simulink model "pglib"  (Simulink 7.0)
settings: Solver=ode45  SolverMode=SingleTasking  StartTime=0.0  StopTime=10.0  RelTol=1e-3  AbsTol=1e-6
(part 1 of 3)
settings Model: Creator=jacobs  LastModifiedBy=lfd  ExtModeAutoUpdateStatusClock=off
settings DataIOCC: LimitDataPoints=off
settings OptimizationCC: BlockReduction=off  BooleanDataType=off
settings DebuggingCC: SaveWithParameterizedLinksMsg=none  SignalResolutionControl=TryResolveAllWithWarning  SolverPrmCheckMsg=none  MultiTaskDSMMsg=warning  MultiTaskCondExecSysMsg=none  StrictBusMsg=None
settings HardwareCC: TargetUnknown=on
settings RTWCC: IncludeERTFirstTime=on
settings GRTTargetCC: TargetFcnLib=ansi_tfl_tmw.mat  ModelReferenceCompliant=off  MatFileLogging=off

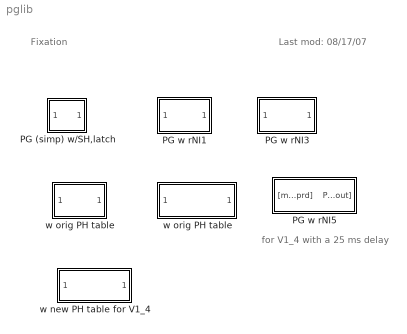
== system pglib ==
  note: Last mod: 08/17/07
  note: Fixation
  note: for V1_4 with a 25 ms delay
  PG (simp) w/SH,latch : Subsystem
      mask Display: disp('PG')
  PG w rNI1 : Subsystem
      mask Display: disp('PG rNI 1\n(2P)')
  PG w rNI3 : Subsystem
      mask Display: disp('PG rNI 1ltnl\n(2P)')
  PG w rNI5 : Subsystem
      mask Display: disp('PG25 rNI V1_4\n(2P)')
  w new PH table for V1_4 : Subsystem
      mask Display: disp('PG rNI V1_4\n(2P)')
  w orig PH table : Subsystem
      mask Display: disp('PG rNI 2\n(2P)')
  "w orig PH table  " : Subsystem
      mask Display: disp('PG rNI V1_4\n(2P)')

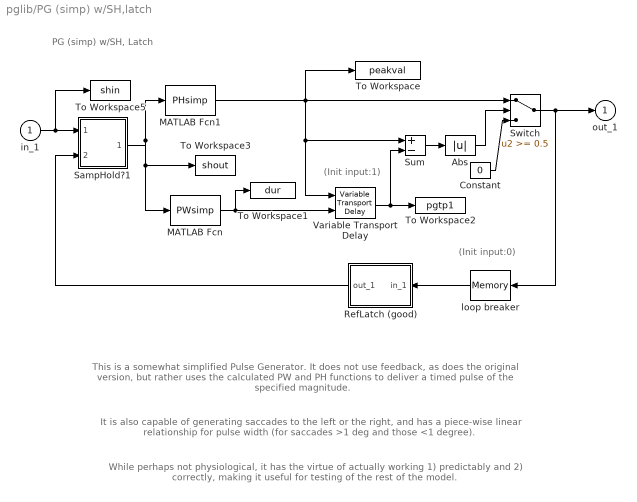
== system pglib/PG (simp) w/SH,latch ==
  note: (Init input:0)
  note: (Init input:1)
  note: PG (simp) w/SH, Latch
  note: This is a somewhat simplified Pulse Generator.  It does not use feedback, as does the
      | original version, but rather uses the calculated PW and PH functions to deliver
      | a timed pulse of the specified magnitude.
  note: It is also capable of generating saccades to the left or the right, and has a piece-wise
      | linear relationship for pulse width (for saccades >1 deg and those <1 degree).
  note: While perhaps not physiological, it has the virtue of actually working
      | 1) predictably and 2) correctly, making it useful for testing of the rest of the model.
  in_1 : Inport  OutDataType=sfix(16)  OutScaling=2^0
  Abs : Abs  SaturateOnIntegerOverflow=on
  Constant : Constant  Value=0  OutDataType=sfix(16)  OutScaling=2^0
  MATLAB Fcn : MATLABFcn  MATLABFcn=PWsimp
      mask Help: u>=1: y=(1.3*abs(u)+12)/1000\nu <1: y=(12*abs(u))/1000
      mask Display: disp('PW\nsimp')
  MATLAB Fcn1 : MATLABFcn  MATLABFcn=PHsimp
      mask Help: u<=0.25: y=0\nu> 0.25:  y = 590*u/(7.5+abs(u))
      mask Display: disp('PH\nsimp')
  RefLatch (good) : Subsystem  Orientation=left  mask{@1=50}
      mask prompts: @1 "Refractory Period (ms)"
      mask help: Refractory Latch
      mask init:
      | delay=@1;
      mask Display: disp('Refract\nLatch')
  SampHold?1 : Subsystem
      mask Display: disp('S&H\n(S=H)\n(H=L)')
  Sum : Sum  Inputs=+-  OutDataType=sfix(16)  OutScaling=2^0  SaturateOnIntegerOverflow=on  InputSameDT=on
  Switch : Switch  Threshold=0.5  SaturateOnIntegerOverflow=on  InputSameDT=on
  To Workspace : ToWorkspace  VariableName=peakval  SaveFormat=Array
      settings: MaxDataPoints=10000
  To Workspace1 : ToWorkspace  VariableName=dur  SaveFormat=Array
      settings: MaxDataPoints=10000
  To Workspace2 : ToWorkspace  VariableName=pgtp1  SaveFormat=Array
      settings: MaxDataPoints=10000
  To Workspace3 : ToWorkspace  VariableName=shout  SaveFormat=Array
      settings: MaxDataPoints=10000
  To Workspace5 : ToWorkspace  VariableName=shin  SaveFormat=Array
      settings: MaxDataPoints=10000
  Variable Transport Delay : VariableTransportDelay  MaximumDelay=10  InitialOutput=1
  loop breaker : Memory  Orientation=left
  out_1 : Outport  OutDataType=sfix(16)  OutScaling=2^0  InitialOutput=0
  wires:
  RefLatch (good)/1(out_1) -> SampHold?1/2(S/H?)
  SampHold?1/1(output) -> To Workspace3/1, MATLAB Fcn/1, MATLAB Fcn1/1
  in_1/1 -> To Workspace5/1, SampHold?1/1(Input)
  MATLAB Fcn1/1 -> To Workspace/1, Sum/1, Variable Transport Delay/1, Switch/1
  Switch/1 -> out_1/1, loop breaker/1
  Constant/1 -> Switch/3
  Variable Transport Delay/1 -> Sum/2, To Workspace2/1
  loop breaker/1 -> RefLatch (good)/1(in_1)
  Abs/1 -> Switch/2
  Sum/1 -> Abs/1
  MATLAB Fcn/1 -> To Workspace1/1, Variable Transport Delay/2

== system pglib/PG w rNI1 ==
  note: (Init input:0)
  note: PG with Resettable NI
  note: The refractory latch prevents the pulse generator from responding to another stimulus until a
      | physiologically acceptable refractory period has elapsed by controlling the "Sample and Hold" block.
  note: Here it is at last!  A pulse generator based on a resettable integrator (look inside the PW
      | block).  The PW function controls the switch, allowing the output of the PH function to pass
      | for the appropriate duration.
  "[mcsprd]" : Inport  OutDataType=sfix(16)  OutScaling=2^0
  Constant1 : Constant  Orientation=up  Value=0  OutDataType=sfix(16)  OutScaling=2^0
  PH funct : MATLABFcn  MATLABFcn=phfn_ss
      mask Display: disp('PH\nfunction')
  PW funct : Subsystem
      mask Display: disp('PW\nfunction')
  RefLatch (Default = 50ms) : Subsystem  Orientation=left  mask{@1=50}
      mask prompts: @1 "Refractory Period (ms)"
      mask help: Refractory Latch
      mask init:
      | delay=@1;
      mask Display: disp('Refract\nLatch')
  SampHold?1 : Subsystem
      mask Display: disp('S=H\nH=L')
  Switch : Switch  Threshold=0.5  SaturateOnIntegerOverflow=on  InputSameDT=on
  loop breaker : Memory  Orientation=left
  PG [pgout] : Outport  OutDataType=sfix(16)  OutScaling=2^0  InitialOutput=0
  wires:
  RefLatch (Default = 50ms)/1(out_1) -> SampHold?1/2(S/H?)
  PH funct/1 -> Switch/1
  PW funct/1(pgw) -> Switch/2
  "[mcsprd]"/1 -> SampHold?1/1(Input)
  SampHold?1/1(output) -> PW funct/1(mcspl), PH funct/1
  loop breaker/1 -> RefLatch (Default = 50ms)/1(in_1)
  Switch/1 -> PG [pgout]/1, loop breaker/1
  Constant1/1 -> Switch/3

== system pglib/PG w rNI3 ==
  note: (Init input:0)
  note: PG with Resettable NI
  note: The refractory latch prevents the pulse generator from responding to another stimulus until a
      | physiologically acceptable refractory period has elapsed by controlling the "Sample and Hold" block.
  note: Here it is at last!  A pulse generator based on a resettable integrator (look inside the PW
      | block).  The PW function controls the switch, allowing the output of the PH function to pass
      | for the appropriate duration.
  "[mcsprd]" : Inport  OutDataType=sfix(16)  OutScaling=2^0
  Constant1 : Constant  Orientation=up  Value=0  OutDataType=sfix(16)  OutScaling=2^0
  PH funct : MATLABFcn  MATLABFcn=phfn_ss
      mask Display: disp('PH\nfunction')
  PW funct : Subsystem
      mask Display: disp('PW\nfunction')
  RefLatch (Default = 50ms) : Subsystem  Orientation=left  mask{@1=50}
      mask prompts: @1 "Refractory Period (ms)"
      mask help: Refractory Latch
      mask init:
      | delay=@1;
      mask Display: disp('Refract\nLatch')
  SampHold?1 : Subsystem
      mask Display: disp('S=H\nH=L')
  Switch : Switch  Threshold=0.5  SaturateOnIntegerOverflow=on  InputSameDT=on
  loop breaker : Memory  Orientation=left
  PG [pgout] : Outport  OutDataType=sfix(16)  OutScaling=2^0  InitialOutput=0
  wires:
  RefLatch (Default = 50ms)/1(out_1) -> SampHold?1/2(S/H?)
  PH funct/1 -> Switch/1
  PW funct/1(pgw) -> Switch/2
  "[mcsprd]"/1 -> SampHold?1/1(Input)
  SampHold?1/1(output) -> PW funct/1(mcspl), PH funct/1
  loop breaker/1 -> RefLatch (Default = 50ms)/1(in_1)
  Switch/1 -> PG [pgout]/1, loop breaker/1
  Constant1/1 -> Switch/3

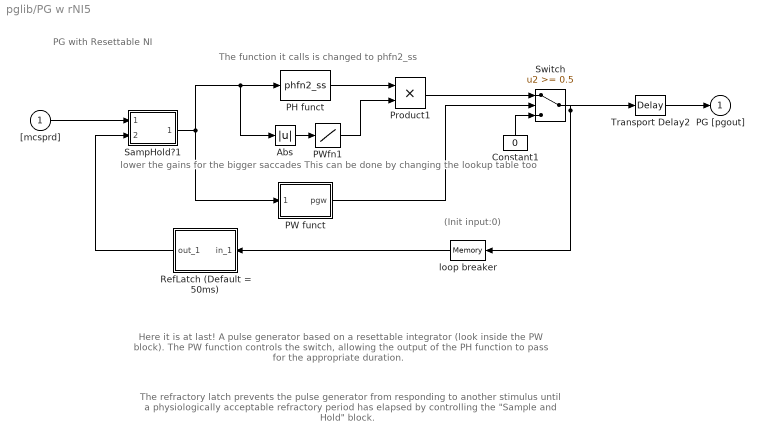
== system pglib/PG w rNI5 ==
  note: (Init input:0)
  note: PG with Resettable NI
  note: The refractory latch prevents the pulse generator from responding to another stimulus until a
      | physiologically acceptable refractory period has elapsed by controlling the "Sample and Hold" block.
  note: Here it is at last!  A pulse generator based on a resettable integrator (look inside the PW
      | block).  The PW function controls the switch, allowing the output of the PH function to pass
      | for the appropriate duration.
  note: lower the gains for the bigger saccades
      | This can be done by changing the lookup table too
  note: The function it calls is changed to phfn2_ss
  "[mcsprd]" : Inport  OutDataType=sfix(16)  OutScaling=2^0
  Abs : Abs  SaturateOnIntegerOverflow=on
  Constant1 : Constant  Orientation=up  Value=0  OutDataType=sfix(16)  OutScaling=2^0
  PH funct : MATLABFcn  MATLABFcn=phfn2_ss
      mask Display: disp('PH\nfunction')
  PW funct : Subsystem
      mask Display: disp('PW\nfunction')
  PWfn1 : Lookup  InputValues=[ 0, 0.1:20, 20:50 ]  Table="[ 0, (0.1:20)*0+1,  (20:50)*0+0.95]"  OutDataType=sfix(16)  OutScaling=2^0  SaturateOnIntegerOverflow=on
  Product1 : Product  OutDataType=sfix(16)  OutScaling=2^0  SaturateOnIntegerOverflow=on  RndMeth=Zero  InputSameDT=on
  RefLatch (Default = 50ms) : Subsystem  Orientation=left  mask{@1=50}
      mask prompts: @1 "Refractory Period (ms)"
      mask help: Refractory Latch
      mask init:
      | delay=@1;
      mask Display: disp('Refract\nLatch')
  SampHold?1 : Subsystem
      mask Display: disp('S=H\nH=L')
  Switch : Switch  Threshold=0.5  SaturateOnIntegerOverflow=on  InputSameDT=on
  Transport Delay2 : TransportDelay  DelayTime=0.025
      mask Display: disp('25ms')
  loop breaker : Memory  Orientation=left
  PG [pgout] : Outport  OutDataType=sfix(16)  OutScaling=2^0  InitialOutput=0
  wires:
  RefLatch (Default = 50ms)/1(out_1) -> SampHold?1/2(S/H?)
  PH funct/1 -> Product1/1
  PW funct/1(pgw) -> Switch/2
  "[mcsprd]"/1 -> SampHold?1/1(Input)
  SampHold?1/1(output) -> PW funct/1(mcspl), PH funct/1, Abs/1
  loop breaker/1 -> RefLatch (Default = 50ms)/1(in_1)
  Switch/1 -> loop breaker/1, Transport Delay2/1
  Constant1/1 -> Switch/3
  Transport Delay2/1 -> PG [pgout]/1
  Product1/1 -> Switch/1
  PWfn1/1 -> Product1/2
  Abs/1 -> PWfn1/1

== system pglib/w new PH table for V1_4 ==
  note: Here it is at last!  A pulse generator based on a resettable integrator (look inside the PW
      | block).  The PW function controls the switch, allowing the output of the PH function to pass
      | for the appropriate duration.
  note: The refractory latch prevents the pulse generator from responding to another stimulus until a
      | physiologically acceptable refractory period has elapsed by controlling the "Sample and Hold" block.
  note: PG with Resettable NI
  note: (Init input:0)
  "[mcsprd]" : Inport  OutDataType=sfix(16)  OutScaling=2^0
  Constant1 : Constant  Orientation=up  Value=0  OutDataType=sfix(16)  OutScaling=2^0
  PH funct : MATLABFcn  MATLABFcn=phfn2_ss
      mask Display: disp('PH\nfunction')
  PW funct : Subsystem
      mask Display: disp('PW\nfunction')
  RefLatch (Default = 50ms) : Subsystem  Orientation=left  mask{@1=50}
      mask prompts: @1 "Refractory Period (ms)"
      mask help: Refractory Latch
      mask init:
      | delay=@1;
      mask Display: disp('Refract\nLatch')
  SampHold?1 : Subsystem
      mask Display: disp('S=H\nH=L')
  Switch : Switch  Threshold=0.5  SaturateOnIntegerOverflow=on  InputSameDT=on
  loop breaker : Memory  Orientation=left
  PG [pgout] : Outport  OutDataType=sfix(16)  OutScaling=2^0  InitialOutput=0
  wires:
  Constant1/1 -> Switch/3
  Switch/1 -> loop breaker/1, PG [pgout]/1
  loop breaker/1 -> RefLatch (Default = 50ms)/1(in_1)
  SampHold?1/1(output) -> PH funct/1, PW funct/1(mcspl)
  "[mcsprd]"/1 -> SampHold?1/1(Input)
  PW funct/1(pgw) -> Switch/2
  PH funct/1 -> Switch/1
  RefLatch (Default = 50ms)/1(out_1) -> SampHold?1/2(S/H?)

== system pglib/w orig PH table ==
  note: (Init input:0)
  note: PG with Resettable NI
  note: The refractory latch prevents the pulse generator from responding to another stimulus until a
      | physiologically acceptable refractory period has elapsed by controlling the "Sample and Hold" block.
  note: Here it is at last!  A pulse generator based on a resettable integrator (look inside the PW
      | block).  The PW function controls the switch, allowing the output of the PH function to pass
      | for the appropriate duration.
  "[mcsprd]" : Inport  OutDataType=sfix(16)  OutScaling=2^0
  Constant1 : Constant  Orientation=up  Value=0  OutDataType=sfix(16)  OutScaling=2^0
  PH funct : MATLABFcn  MATLABFcn=phfn_ss
      mask Display: disp('PH\nfunction')
  PW funct : Subsystem
      mask Display: disp('PW\nfunction')
  RefLatch (Default = 50ms) : Subsystem  Orientation=left  mask{@1=50}
      mask prompts: @1 "Refractory Period (ms)"
      mask help: Refractory Latch
      mask init:
      | delay=@1;
      mask Display: disp('Refract\nLatch')
  SampHold?1 : Subsystem
      mask Display: disp('S=H\nH=L')
  Switch : Switch  Threshold=0.5  SaturateOnIntegerOverflow=on  InputSameDT=on
  loop breaker : Memory  Orientation=left
  PG [pgout] : Outport  OutDataType=sfix(16)  OutScaling=2^0  InitialOutput=0
  wires:
  RefLatch (Default = 50ms)/1(out_1) -> SampHold?1/2(S/H?)
  PH funct/1 -> Switch/1
  PW funct/1(pgw) -> Switch/2
  "[mcsprd]"/1 -> SampHold?1/1(Input)
  SampHold?1/1(output) -> PW funct/1(mcspl), PH funct/1
  loop breaker/1 -> RefLatch (Default = 50ms)/1(in_1)
  Switch/1 -> PG [pgout]/1, loop breaker/1
  Constant1/1 -> Switch/3

== system pglib/w orig PH table   ==
  note: Here it is at last!  A pulse generator based on a resettable integrator (look inside the PW
      | block).  The PW function controls the switch, allowing the output of the PH function to pass
      | for the appropriate duration.
  note: The refractory latch prevents the pulse generator from responding to another stimulus until a
      | physiologically acceptable refractory period has elapsed by controlling the "Sample and Hold" block.
  note: PG with Resettable NI
  note: (Init input:0)
  "[mcsprd]" : Inport  OutDataType=sfix(16)  OutScaling=2^0
  Constant1 : Constant  Orientation=up  Value=0  OutDataType=sfix(16)  OutScaling=2^0
  PH funct : MATLABFcn  MATLABFcn=phfn_ss
      mask Display: disp('PH\nfunction')
  PW funct : Subsystem
      mask Display: disp('PW\nfunction')
  RefLatch (Default = 50ms) : Subsystem  Orientation=left  mask{@1=50}
      mask prompts: @1 "Refractory Period (ms)"
      mask help: Refractory Latch
      mask init:
      | delay=@1;
      mask Display: disp('Refract\nLatch')
  SampHold?1 : Subsystem
      mask Display: disp('S=H\nH=L')
  Switch : Switch  Threshold=0.5  SaturateOnIntegerOverflow=on  InputSameDT=on
  loop breaker : Memory  Orientation=left
  PG [pgout] : Outport  OutDataType=sfix(16)  OutScaling=2^0  InitialOutput=0
  wires:
  Constant1/1 -> Switch/3
  Switch/1 -> loop breaker/1, PG [pgout]/1
  loop breaker/1 -> RefLatch (Default = 50ms)/1(in_1)
  SampHold?1/1(output) -> PH funct/1, PW funct/1(mcspl)
  "[mcsprd]"/1 -> SampHold?1/1(Input)
  PW funct/1(pgw) -> Switch/2
  PH funct/1 -> Switch/1
  RefLatch (Default = 50ms)/1(out_1) -> SampHold?1/2(S/H?)

== system pglib/PG (simp) w/SH,latch/RefLatch (good) ==
  note: It's a cheap trick, but it seems to work:
  note: The falling edge" block's output becomes DISABLED upon
      | detection of the END of the input pulse, and remains
      | so until the refractory period of rp milliseconds has elapsed.
  note: By ANDing these outputs, we get a signal that is DISABLED
      | starting with the beginning of the input pulse, and remains so until
      | rp milliseconds after the termination of the pulse.
  note: The "NOT" gate outputs a DISABLE signal whenever there is any
      | input, so that there can be no response.
  in_1 : Inport  OutDataType=sfix(16)  OutScaling=2^0
  Abs : Abs  SaturateOnIntegerOverflow=on
  Logical Operator : Logic
  Logical Operator1 : Logic  Operator=NOT  Inputs=1
  trailing edge : Subsystem
      mask Display: disp('Refract\nLatch (te)')
  out_1 : Outport  OutDataType=sfix(16)  OutScaling=2^0  InitialOutput=0
  wires:
  Logical Operator/1 -> out_1/1
  Logical Operator1/1 -> Logical Operator/1
  trailing edge/1(out_1) -> Logical Operator/2
  Abs/1 -> trailing edge/1(in_1), Logical Operator1/1
  in_1/1 -> Abs/1

== system pglib/PG (simp) w/SH,latch/SampHold?1 ==
  note: When "S/H?" is HIGH, then "Input" is switched directly to the
      | output ("sample").  When "S/H?" is LOW, the current output is
      | maintained ("hold").
  Input : Inport  OutDataType=sfix(16)  OutScaling=2^0
  S/H? : Inport  Port=2  OutDataType=sfix(16)  OutScaling=2^0
  Memory : Memory  Orientation=left
  Sign : Subsystem
      mask Type: Sign
      mask Description: y = sign(x)
      mask Help: Sign Function:\n\t\t\ty = 1 if x > 0\n\t\t\ty = 0 if x = 0\n\t\t\ty = -1 if x < 0
      mask Display: plot(-50,-50,50,50,[-50,50],[0,0],[0,0],[-50,50],[-40,0],[-30,-30],[0,40],[30,30])
  Switch2 : Switch  Threshold=0.5  SaturateOnIntegerOverflow=on  InputSameDT=on
  output : Outport  OutDataType=sfix(16)  OutScaling=2^0  InitialOutput=0
  wires:
  Memory/1 -> Switch2/3
  Switch2/1 -> Memory/1, output/1
  Input/1 -> Switch2/1
  Sign/1(out_1) -> Switch2/2
  S/H?/1 -> Sign/1(in_1)

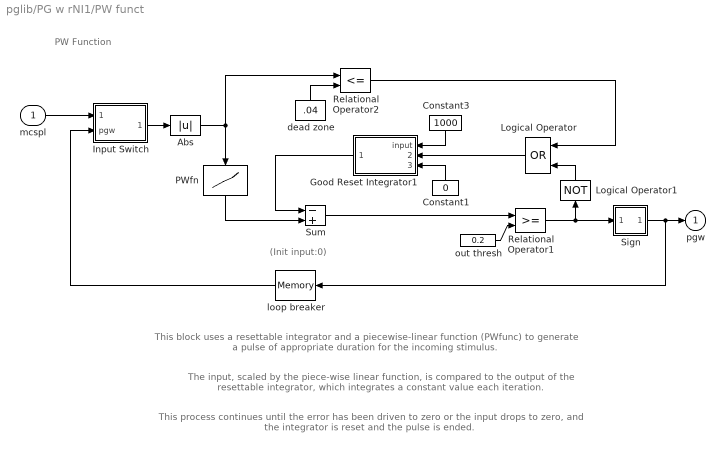
== system pglib/PG w rNI1/PW funct ==
  note: PW Function
  note: (Init input:0)
  note: This block uses a resettable integrator and a piecewise-linear function (PWfunc) to generate
      | a pulse of appropriate duration for the incoming stimulus.
  note: The input, scaled by the piece-wise linear function, is compared to the output of the
      | resettable integrator, which integrates a constant value each iteration.
  note: This process continues until the error has been driven to zero or the input drops to zero,
      | and the integrator is reset and the pulse is ended.
  mcspl : Inport  OutDataType=sfix(16)  OutScaling=2^0
  Abs : Abs  SaturateOnIntegerOverflow=on
  Constant1 : Constant  Orientation=up  Value=0  OutDataType=sfix(16)  OutScaling=2^0
  Constant3 : Constant  Orientation=down  Value=1000  OutDataType=sfix(16)  OutScaling=2^0
  Good Reset Integrator1 : Subsystem  Orientation=left
      mask Display: disp('Resettable\nNI')
  Input Switch : Subsystem
      mask Display: disp('Input\nSwitch')
  Logical Operator : Logic  Orientation=left  Operator=OR
  Logical Operator1 : Logic  Orientation=up  Operator=NOT  Inputs=1
  PWfn : Lookup  Orientation=down  InputValues=[ 0, 0.1:5, 5:10, 10:50 ]  Table="[ 0, (0.1:5)*0+15,  (5:10)*1+10,  (10:50)*2]"  OutDataType=sfix(16)  OutScaling=2^0  SaturateOnIntegerOverflow=on
  Relational Operator1 : RelationalOperator  InputSameDT=on
  Relational Operator2 : RelationalOperator  Operator=<=  InputSameDT=on
  Sign : Subsystem
      mask Type: Sign
      mask Description: y = sign(x)
      mask Help: Sign Function:\n\t\t\ty = 1 if x > 0\n\t\t\ty = 0 if x = 0\n\t\t\ty = -1 if x < 0
      mask Display: plot(-50,-50,50,50,[-50,50],[0,0],[0,0],[-50,50],[-40,0],[-30,-30],[0,40],[30,30])
  Sum : Sum  Inputs=-+  OutDataType=sfix(16)  OutScaling=2^0  SaturateOnIntegerOverflow=on  InputSameDT=on
  dead zone : Constant  Orientation=up  Value=.04  OutDataType=sfix(16)  OutScaling=2^0
  loop breaker : Memory  Orientation=left
  out thresh : Constant  Value=0.2  OutDataType=sfix(16)  OutScaling=2^0
  pgw : Outport  OutDataType=sfix(16)  OutScaling=2^0  InitialOutput=0
  wires:
  loop breaker/1 -> Input Switch/2(pgw)
  Relational Operator2/1 -> Logical Operator/1
  dead zone/1 -> Relational Operator2/2
  Good Reset Integrator1/1(out_1) -> Sum/1
  Logical Operator/1 -> Good Reset Integrator1/2(reset?)
  Sum/1 -> Relational Operator1/1
  PWfn/1 -> Sum/2
  Abs/1 -> Relational Operator2/1, PWfn/1
  Sign/1(out_1) -> loop breaker/1, pgw/1
  mcspl/1 -> Input Switch/1(mcspl)
  Input Switch/1(mcsw) -> Abs/1
  out thresh/1 -> Relational Operator1/2
  Constant1/1 -> Good Reset Integrator1/3(initial condition)
  Constant3/1 -> Good Reset Integrator1/1(input)
  Relational Operator1/1 -> Sign/1(in_1), Logical Operator1/1
  Logical Operator1/1 -> Logical Operator/2

== system pglib/PG w rNI1/RefLatch (Default = 50ms) ==
  note: The "NOT" gate outputs a DISABLE signal whenever there is any
      | input, so that there can be no response.
  note: By ANDing these outputs, we get a signal that is DISABLED
      | starting with the beginning of the input pulse, and remains so until
      | rp milliseconds after the termination of the pulse.
  note: The falling edge" block's output becomes DISABLED upon
      | detection of the END of the input pulse, and remains
      | so until the refractory period of rp milliseconds has elapsed.
  note: It's a cheap trick, but it seems to work:
  in_1 : Inport  OutDataType=sfix(16)  OutScaling=2^0
  Abs : Abs  SaturateOnIntegerOverflow=on
  Logical Operator : Logic
  Logical Operator1 : Logic  Operator=NOT  Inputs=1
  trailing edge : Subsystem
      mask Display: disp('Refract\nLatch (te)')
  out_1 : Outport  OutDataType=sfix(16)  OutScaling=2^0  InitialOutput=0
  wires:
  in_1/1 -> Abs/1
  Abs/1 -> trailing edge/1(in_1), Logical Operator1/1
  trailing edge/1(out_1) -> Logical Operator/2
  Logical Operator1/1 -> Logical Operator/1
  Logical Operator/1 -> out_1/1

== system pglib/PG w rNI1/SampHold?1 ==
  note: When "S/H?" is HIGH, then "Input" is switched directly to the
      | output ("sample").  When "S/H?" is LOW, the current output is
      | maintained ("hold").
  Input : Inport  OutDataType=sfix(16)  OutScaling=2^0
  S/H? : Inport  Port=2  OutDataType=sfix(16)  OutScaling=2^0
  Memory : Memory  Orientation=left
  Sign : Subsystem
      mask Type: Sign
      mask Description: y = sign(x)
      mask Help: Sign Function:\n\t\t\ty = 1 if x > 0\n\t\t\ty = 0 if x = 0\n\t\t\ty = -1 if x < 0
      mask Display: plot(-50,-50,50,50,[-50,50],[0,0],[0,0],[-50,50],[-40,0],[-30,-30],[0,40],[30,30])
  Switch2 : Switch  Threshold=0.5  SaturateOnIntegerOverflow=on  InputSameDT=on
  output : Outport  OutDataType=sfix(16)  OutScaling=2^0  InitialOutput=0
  wires:
  Memory/1 -> Switch2/3
  Switch2/1 -> Memory/1, output/1
  Input/1 -> Switch2/1
  Sign/1(out_1) -> Switch2/2
  S/H?/1 -> Sign/1(in_1)

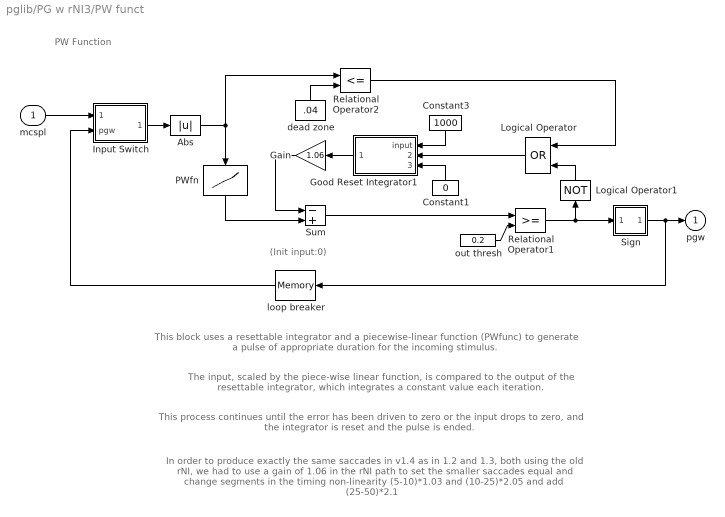
== system pglib/PG w rNI3/PW funct ==
  note: In order to produce exactly the same saccades in v1.4 as in 1.2 and 1.3, both using the old rNI,
      | we had to use a gain of 1.06 in the rNI path to set the smaller saccades equal
      | and change segments in the timing non-linearity (5-10)*1.03 and  (10-25)*2.05 and add (25-50)*2.1
  note: PW Function
  note: (Init input:0)
  note: This block uses a resettable integrator and a piecewise-linear function (PWfunc) to generate
      | a pulse of appropriate duration for the incoming stimulus.
  note: The input, scaled by the piece-wise linear function, is compared to the output of the
      | resettable integrator, which integrates a constant value each iteration.
  note: This process continues until the error has been driven to zero or the input drops to zero,
      | and the integrator is reset and the pulse is ended.
  mcspl : Inport  OutDataType=sfix(16)  OutScaling=2^0
  Abs : Abs  SaturateOnIntegerOverflow=on
  Constant1 : Constant  Orientation=up  Value=0  OutDataType=sfix(16)  OutScaling=2^0
  Constant3 : Constant  Orientation=down  Value=1000  OutDataType=sfix(16)  OutScaling=2^0
  Gain : Gain  Orientation=left  Gain=1.06  ParameterDataType=sfix(16)  ParameterScaling=2^0  OutDataType=sfix(16)  OutScaling=2^0
  Good Reset Integrator1 : Subsystem  Orientation=left
      mask Display: disp('Resettable\nNI')
  Input Switch : Subsystem
      mask Display: disp('Input\nSwitch')
  Logical Operator : Logic  Orientation=left  Operator=OR
  Logical Operator1 : Logic  Orientation=up  Operator=NOT  Inputs=1
  PWfn : Lookup  Orientation=down  InputValues=[ 0, 0.1:5, 5:10, 10:25, 25:50 ]  Table="[ 0, (0.1:5)*0+15,  (5:10)*1.03+10, (10:25)*2.05, (25:50)*2.1]"  OutDataType=sfix(16)  OutScaling=2^0  SaturateOnIntegerOverflow=on
  Relational Operator1 : RelationalOperator  InputSameDT=on
  Relational Operator2 : RelationalOperator  Operator=<=  InputSameDT=on
  Sign : Subsystem
      mask Type: Sign
      mask Description: y = sign(x)
      mask Help: Sign Function:\n\t\t\ty = 1 if x > 0\n\t\t\ty = 0 if x = 0\n\t\t\ty = -1 if x < 0
      mask Display: plot(-50,-50,50,50,[-50,50],[0,0],[0,0],[-50,50],[-40,0],[-30,-30],[0,40],[30,30])
  Sum : Sum  Inputs=-+  OutDataType=sfix(16)  OutScaling=2^0  SaturateOnIntegerOverflow=on  InputSameDT=on
  dead zone : Constant  Orientation=up  Value=.04  OutDataType=sfix(16)  OutScaling=2^0
  loop breaker : Memory  Orientation=left
  out thresh : Constant  Value=0.2  OutDataType=sfix(16)  OutScaling=2^0
  pgw : Outport  OutDataType=sfix(16)  OutScaling=2^0  InitialOutput=0
  wires:
  Gain/1 -> Sum/1
  loop breaker/1 -> Input Switch/2(pgw)
  Relational Operator2/1 -> Logical Operator/1
  dead zone/1 -> Relational Operator2/2
  Good Reset Integrator1/1(out_1) -> Gain/1
  Logical Operator/1 -> Good Reset Integrator1/2(reset?)
  Sum/1 -> Relational Operator1/1
  PWfn/1 -> Sum/2
  Abs/1 -> Relational Operator2/1, PWfn/1
  Sign/1(out_1) -> loop breaker/1, pgw/1
  mcspl/1 -> Input Switch/1(mcspl)
  Input Switch/1(mcsw) -> Abs/1
  out thresh/1 -> Relational Operator1/2
  Constant1/1 -> Good Reset Integrator1/3(initial condition)
  Constant3/1 -> Good Reset Integrator1/1(input)
  Relational Operator1/1 -> Sign/1(in_1), Logical Operator1/1
  Logical Operator1/1 -> Logical Operator/2

== system pglib/PG w rNI3/RefLatch (Default = 50ms) ==
  note: The "NOT" gate outputs a DISABLE signal whenever there is any
      | input, so that there can be no response.
  note: By ANDing these outputs, we get a signal that is DISABLED
      | starting with the beginning of the input pulse, and remains so until
      | rp milliseconds after the termination of the pulse.
  note: The falling edge" block's output becomes DISABLED upon
      | detection of the END of the input pulse, and remains
      | so until the refractory period of rp milliseconds has elapsed.
  note: It's a cheap trick, but it seems to work:
  in_1 : Inport  OutDataType=sfix(16)  OutScaling=2^0
  Abs : Abs  SaturateOnIntegerOverflow=on
  Logical Operator : Logic
  Logical Operator1 : Logic  Operator=NOT  Inputs=1
  trailing edge : Subsystem
      mask Display: disp('Refract\nLatch (te)')
  out_1 : Outport  OutDataType=sfix(16)  OutScaling=2^0  InitialOutput=0
  wires:
  in_1/1 -> Abs/1
  Abs/1 -> trailing edge/1(in_1), Logical Operator1/1
  trailing edge/1(out_1) -> Logical Operator/2
  Logical Operator1/1 -> Logical Operator/1
  Logical Operator/1 -> out_1/1

== system pglib/PG w rNI3/SampHold?1 ==
  note: When "S/H?" is HIGH, then "Input" is switched directly to the
      | output ("sample").  When "S/H?" is LOW, the current output is
      | maintained ("hold").
  Input : Inport  OutDataType=sfix(16)  OutScaling=2^0
  S/H? : Inport  Port=2  OutDataType=sfix(16)  OutScaling=2^0
  Memory : Memory  Orientation=left
  Sign : Subsystem
      mask Type: Sign
      mask Description: y = sign(x)
      mask Help: Sign Function:\n\t\t\ty = 1 if x > 0\n\t\t\ty = 0 if x = 0\n\t\t\ty = -1 if x < 0
      mask Display: plot(-50,-50,50,50,[-50,50],[0,0],[0,0],[-50,50],[-40,0],[-30,-30],[0,40],[30,30])
  Switch2 : Switch  Threshold=0.5  SaturateOnIntegerOverflow=on  InputSameDT=on
  output : Outport  OutDataType=sfix(16)  OutScaling=2^0  InitialOutput=0
  wires:
  Memory/1 -> Switch2/3
  Switch2/1 -> Memory/1, output/1
  Input/1 -> Switch2/1
  Sign/1(out_1) -> Switch2/2
  S/H?/1 -> Sign/1(in_1)

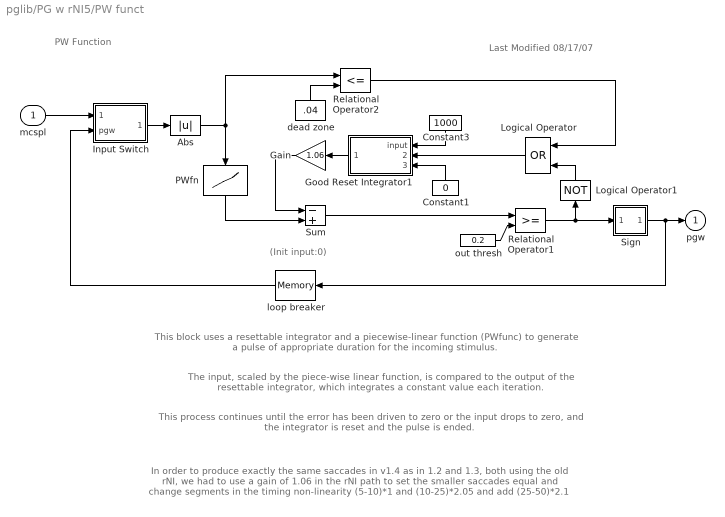
== system pglib/PG w rNI5/PW funct ==
  note: In order to produce exactly the same saccades in v1.4 as in 1.2 and 1.3, both using the old rNI,
      | we had to use a gain of 1.06 in the rNI path to set the smaller saccades equal
      | and change segments in the timing non-linearity (5-10)*1 and  (10-25)*2.05 and add (25-50)*2.1
  note: Last Modified
      | 08/17/07
  note: PW Function
  note: (Init input:0)
  note: This block uses a resettable integrator and a piecewise-linear function (PWfunc) to generate
      | a pulse of appropriate duration for the incoming stimulus.
  note: The input, scaled by the piece-wise linear function, is compared to the output of the
      | resettable integrator, which integrates a constant value each iteration.
  note: This process continues until the error has been driven to zero or the input drops to zero,
      | and the integrator is reset and the pulse is ended.
  mcspl : Inport  OutDataType=sfix(16)  OutScaling=2^0
  Abs : Abs  SaturateOnIntegerOverflow=on
  Constant1 : Constant  Orientation=up  Value=0  OutDataType=sfix(16)  OutScaling=2^0
  Constant3 : Constant  Orientation=down  Value=1000  OutDataType=sfix(16)  OutScaling=2^0
  Gain : Gain  Orientation=left  Gain=1.06  ParameterDataType=sfix(16)  ParameterScaling=2^0  OutDataType=sfix(16)  OutScaling=2^0
  Good Reset Integrator1 : Subsystem  Orientation=left
      mask Display: disp('Resettable\nNI')
  Input Switch : Subsystem
      mask Display: disp('Input\nSwitch')
  Logical Operator : Logic  Orientation=left  Operator=OR
  Logical Operator1 : Logic  Orientation=up  Operator=NOT  Inputs=1
  PWfn : Lookup  Orientation=down  InputValues=[ 0, 0.1:5, 5:10, 10:15, 15:25, 25:50 ]  Table="[ 0, (0.1:5)*0+15,  (5:10)*1+10,  (10:15)*2.0, (15:25)*2.05,  (25:50)*2.1]"  OutDataType=sfix(16)  OutScaling=2^0  SaturateOnIntegerOverflow=on
  Relational Operator1 : RelationalOperator  InputSameDT=on
  Relational Operator2 : RelationalOperator  Operator=<=  InputSameDT=on
  Sign : Subsystem
      mask Type: Sign
      mask Description: y = sign(x)
      mask Help: Sign Function:\n\t\t\ty = 1 if x > 0\n\t\t\ty = 0 if x = 0\n\t\t\ty = -1 if x < 0
      mask Display: plot(-50,-50,50,50,[-50,50],[0,0],[0,0],[-50,50],[-40,0],[-30,-30],[0,40],[30,30])
  Sum : Sum  Inputs=-+  OutDataType=sfix(16)  OutScaling=2^0  SaturateOnIntegerOverflow=on  InputSameDT=on
  dead zone : Constant  Orientation=up  Value=.04  OutDataType=sfix(16)  OutScaling=2^0
  loop breaker : Memory  Orientation=left
  out thresh : Constant  Value=0.2  OutDataType=sfix(16)  OutScaling=2^0
  pgw : Outport  OutDataType=sfix(16)  OutScaling=2^0  InitialOutput=0
  wires:
  Gain/1 -> Sum/1
  loop breaker/1 -> Input Switch/2(pgw)
  Relational Operator2/1 -> Logical Operator/1
  dead zone/1 -> Relational Operator2/2
  Good Reset Integrator1/1(out_1) -> Gain/1
  Logical Operator/1 -> Good Reset Integrator1/2(reset?)
  Sum/1 -> Relational Operator1/1
  PWfn/1 -> Sum/2
  Abs/1 -> Relational Operator2/1, PWfn/1
  Sign/1(out_1) -> loop breaker/1, pgw/1
  mcspl/1 -> Input Switch/1(mcspl)
  Input Switch/1(mcsw) -> Abs/1
  out thresh/1 -> Relational Operator1/2
  Constant1/1 -> Good Reset Integrator1/3(initial condition)
  Constant3/1 -> Good Reset Integrator1/1(input)
  Relational Operator1/1 -> Sign/1(in_1), Logical Operator1/1
  Logical Operator1/1 -> Logical Operator/2

== system pglib/PG w rNI5/RefLatch (Default = 50ms) ==
  note: The "NOT" gate outputs a DISABLE signal whenever there is any
      | input, so that there can be no response.
  note: By ANDing these outputs, we get a signal that is DISABLED
      | starting with the beginning of the input pulse, and remains so until
      | rp milliseconds after the termination of the pulse.
  note: The falling edge" block's output becomes DISABLED upon
      | detection of the END of the input pulse, and remains
      | so until the refractory period of rp milliseconds has elapsed.
  note: It's a cheap trick, but it seems to work:
  in_1 : Inport  OutDataType=sfix(16)  OutScaling=2^0
  Abs : Abs  SaturateOnIntegerOverflow=on
  Logical Operator : Logic
  Logical Operator1 : Logic  Operator=NOT  Inputs=1
  trailing edge : Subsystem
      mask Display: disp('Refract\nLatch (te)')
  out_1 : Outport  OutDataType=sfix(16)  OutScaling=2^0  InitialOutput=0
  wires:
  in_1/1 -> Abs/1
  Abs/1 -> trailing edge/1(in_1), Logical Operator1/1
  trailing edge/1(out_1) -> Logical Operator/2
  Logical Operator1/1 -> Logical Operator/1
  Logical Operator/1 -> out_1/1

== system pglib/PG w rNI5/SampHold?1 ==
  note: When "S/H?" is HIGH, then "Input" is switched directly to the
      | output ("sample").  When "S/H?" is LOW, the current output is
      | maintained ("hold").
  Input : Inport  OutDataType=sfix(16)  OutScaling=2^0
  S/H? : Inport  Port=2  OutDataType=sfix(16)  OutScaling=2^0
  Memory : Memory  Orientation=left
  Sign : Subsystem
      mask Type: Sign
      mask Description: y = sign(x)
      mask Help: Sign Function:\n\t\t\ty = 1 if x > 0\n\t\t\ty = 0 if x = 0\n\t\t\ty = -1 if x < 0
      mask Display: plot(-50,-50,50,50,[-50,50],[0,0],[0,0],[-50,50],[-40,0],[-30,-30],[0,40],[30,30])
  Switch2 : Switch  Threshold=0.5  SaturateOnIntegerOverflow=on  InputSameDT=on
  output : Outport  OutDataType=sfix(16)  OutScaling=2^0  InitialOutput=0
  wires:
  Memory/1 -> Switch2/3
  Switch2/1 -> Memory/1, output/1
  Input/1 -> Switch2/1
  Sign/1(out_1) -> Switch2/2
  S/H?/1 -> Sign/1(in_1)

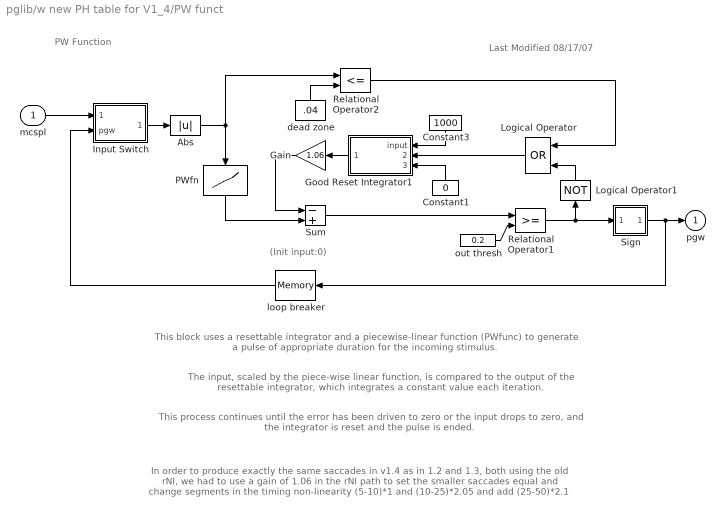
== system pglib/w new PH table for V1_4/PW funct ==
  note: This process continues until the error has been driven to zero or the input drops to zero,
      | and the integrator is reset and the pulse is ended.
  note: The input, scaled by the piece-wise linear function, is compared to the output of the
      | resettable integrator, which integrates a constant value each iteration.
  note: This block uses a resettable integrator and a piecewise-linear function (PWfunc) to generate
      | a pulse of appropriate duration for the incoming stimulus.
  note: (Init input:0)
  note: PW Function
  note: Last Modified
      | 08/17/07
  note: In order to produce exactly the same saccades in v1.4 as in 1.2 and 1.3, both using the old rNI,
      | we had to use a gain of 1.06 in the rNI path to set the smaller saccades equal
      | and change segments in the timing non-linearity (5-10)*1 and  (10-25)*2.05 and add (25-50)*2.1
  mcspl : Inport  OutDataType=sfix(16)  OutScaling=2^0
  Abs : Abs  SaturateOnIntegerOverflow=on
  Constant1 : Constant  Orientation=up  Value=0  OutDataType=sfix(16)  OutScaling=2^0
  Constant3 : Constant  Orientation=down  Value=1000  OutDataType=sfix(16)  OutScaling=2^0
  Gain : Gain  Orientation=left  Gain=1.06  ParameterDataType=sfix(16)  ParameterScaling=2^0  OutDataType=sfix(16)  OutScaling=2^0
  Good Reset Integrator1 : Subsystem  Orientation=left
      mask Display: disp('Resettable\nNI')
  Input Switch : Subsystem
      mask Display: disp('Input\nSwitch')
  Logical Operator : Logic  Orientation=left  Operator=OR
  Logical Operator1 : Logic  Orientation=up  Operator=NOT  Inputs=1
  PWfn : Lookup  Orientation=down  InputValues=[ 0, 0.1:5, 5:10, 10:25, 25:50 ]  Table="[ 0, (0.1:5)*0+15,  (5:10)*1+10,  (10:25)*2.05,  (25:50)*2.1]"  OutDataType=sfix(16)  OutScaling=2^0  SaturateOnIntegerOverflow=on
  Relational Operator1 : RelationalOperator  InputSameDT=on
  Relational Operator2 : RelationalOperator  Operator=<=  InputSameDT=on
  Sign : Subsystem
      mask Type: Sign
      mask Description: y = sign(x)
      mask Help: Sign Function:\n\t\t\ty = 1 if x > 0\n\t\t\ty = 0 if x = 0\n\t\t\ty = -1 if x < 0
      mask Display: plot(-50,-50,50,50,[-50,50],[0,0],[0,0],[-50,50],[-40,0],[-30,-30],[0,40],[30,30])
  Sum : Sum  Inputs=-+  OutDataType=sfix(16)  OutScaling=2^0  SaturateOnIntegerOverflow=on  InputSameDT=on
  dead zone : Constant  Orientation=up  Value=.04  OutDataType=sfix(16)  OutScaling=2^0
  loop breaker : Memory  Orientation=left
  out thresh : Constant  Value=0.2  OutDataType=sfix(16)  OutScaling=2^0
  pgw : Outport  OutDataType=sfix(16)  OutScaling=2^0  InitialOutput=0
  wires:
  Logical Operator1/1 -> Logical Operator/2
  Relational Operator1/1 -> Logical Operator1/1, Sign/1(in_1)
  Constant3/1 -> Good Reset Integrator1/1(input)
  Constant1/1 -> Good Reset Integrator1/3(initial condition)
  out thresh/1 -> Relational Operator1/2
  Input Switch/1(mcsw) -> Abs/1
  mcspl/1 -> Input Switch/1(mcspl)
  Sign/1(out_1) -> pgw/1, loop breaker/1
  Abs/1 -> PWfn/1, Relational Operator2/1
  PWfn/1 -> Sum/2
  Sum/1 -> Relational Operator1/1
  Logical Operator/1 -> Good Reset Integrator1/2(reset?)
  Good Reset Integrator1/1(out_1) -> Gain/1
  dead zone/1 -> Relational Operator2/2
  Relational Operator2/1 -> Logical Operator/1
  loop breaker/1 -> Input Switch/2(pgw)
  Gain/1 -> Sum/1

== system pglib/w new PH table for V1_4/RefLatch (Default = 50ms) ==
  note: It's a cheap trick, but it seems to work:
  note: The falling edge" block's output becomes DISABLED upon
      | detection of the END of the input pulse, and remains
      | so until the refractory period of rp milliseconds has elapsed.
  note: By ANDing these outputs, we get a signal that is DISABLED
      | starting with the beginning of the input pulse, and remains so until
      | rp milliseconds after the termination of the pulse.
  note: The "NOT" gate outputs a DISABLE signal whenever there is any
      | input, so that there can be no response.
  in_1 : Inport  OutDataType=sfix(16)  OutScaling=2^0
  Abs : Abs  SaturateOnIntegerOverflow=on
  Logical Operator : Logic
  Logical Operator1 : Logic  Operator=NOT  Inputs=1
  trailing edge : Subsystem
      mask Display: disp('Refract\nLatch (te)')
  out_1 : Outport  OutDataType=sfix(16)  OutScaling=2^0  InitialOutput=0
  wires:
  Logical Operator/1 -> out_1/1
  Logical Operator1/1 -> Logical Operator/1
  trailing edge/1(out_1) -> Logical Operator/2
  Abs/1 -> Logical Operator1/1, trailing edge/1(in_1)
  in_1/1 -> Abs/1

== system pglib/w new PH table for V1_4/SampHold?1 ==
  note: When "S/H?" is HIGH, then "Input" is switched directly to the
      | output ("sample").  When "S/H?" is LOW, the current output is
      | maintained ("hold").
  Input : Inport  OutDataType=sfix(16)  OutScaling=2^0
  S/H? : Inport  Port=2  OutDataType=sfix(16)  OutScaling=2^0
  Memory : Memory  Orientation=left
  Sign : Subsystem
      mask Type: Sign
      mask Description: y = sign(x)
      mask Help: Sign Function:\n\t\t\ty = 1 if x > 0\n\t\t\ty = 0 if x = 0\n\t\t\ty = -1 if x < 0
      mask Display: plot(-50,-50,50,50,[-50,50],[0,0],[0,0],[-50,50],[-40,0],[-30,-30],[0,40],[30,30])
  Switch2 : Switch  Threshold=0.5  SaturateOnIntegerOverflow=on  InputSameDT=on
  output : Outport  OutDataType=sfix(16)  OutScaling=2^0  InitialOutput=0
  wires:
  S/H?/1 -> Sign/1(in_1)
  Sign/1(out_1) -> Switch2/2
  Input/1 -> Switch2/1
  Switch2/1 -> output/1, Memory/1
  Memory/1 -> Switch2/3

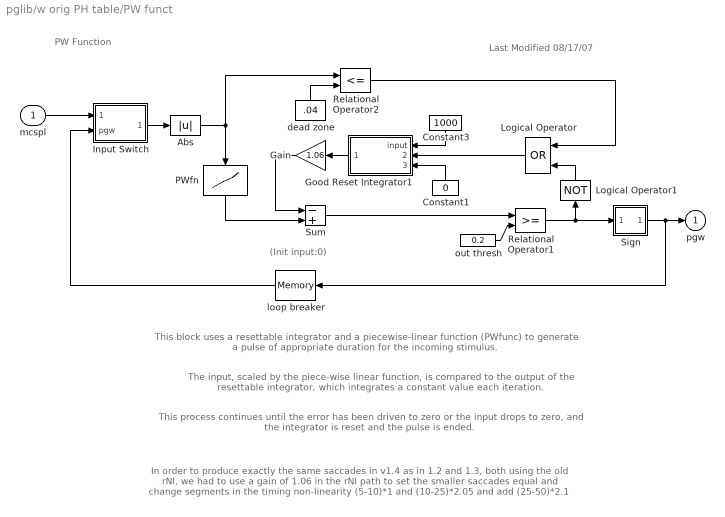
== system pglib/w orig PH table/PW funct ==
  note: In order to produce exactly the same saccades in v1.4 as in 1.2 and 1.3, both using the old rNI,
      | we had to use a gain of 1.06 in the rNI path to set the smaller saccades equal
      | and change segments in the timing non-linearity (5-10)*1 and  (10-25)*2.05 and add (25-50)*2.1
  note: Last Modified
      | 08/17/07
  note: PW Function
  note: (Init input:0)
  note: This block uses a resettable integrator and a piecewise-linear function (PWfunc) to generate
      | a pulse of appropriate duration for the incoming stimulus.
  note: The input, scaled by the piece-wise linear function, is compared to the output of the
      | resettable integrator, which integrates a constant value each iteration.
  note: This process continues until the error has been driven to zero or the input drops to zero,
      | and the integrator is reset and the pulse is ended.
  mcspl : Inport  OutDataType=sfix(16)  OutScaling=2^0
  Abs : Abs  SaturateOnIntegerOverflow=on
  Constant1 : Constant  Orientation=up  Value=0  OutDataType=sfix(16)  OutScaling=2^0
  Constant3 : Constant  Orientation=down  Value=1000  OutDataType=sfix(16)  OutScaling=2^0
  Gain : Gain  Orientation=left  Gain=1.06  ParameterDataType=sfix(16)  ParameterScaling=2^0  OutDataType=sfix(16)  OutScaling=2^0
  Good Reset Integrator1 : Subsystem  Orientation=left
      mask Display: disp('Resettable\nNI')
  Input Switch : Subsystem
      mask Display: disp('Input\nSwitch')
  Logical Operator : Logic  Orientation=left  Operator=OR
  Logical Operator1 : Logic  Orientation=up  Operator=NOT  Inputs=1
  PWfn : Lookup  Orientation=down  InputValues=[ 0, 0.1:5, 5:10, 10:25, 25:50 ]  Table="[ 0, (0.1:5)*0+15,  (5:10)*1+10,  (10:25)*2.05,  (25:50)*2.1]"  OutDataType=sfix(16)  OutScaling=2^0  SaturateOnIntegerOverflow=on
  Relational Operator1 : RelationalOperator  InputSameDT=on
  Relational Operator2 : RelationalOperator  Operator=<=  InputSameDT=on
  Sign : Subsystem
      mask Type: Sign
      mask Description: y = sign(x)
      mask Help: Sign Function:\n\t\t\ty = 1 if x > 0\n\t\t\ty = 0 if x = 0\n\t\t\ty = -1 if x < 0
      mask Display: plot(-50,-50,50,50,[-50,50],[0,0],[0,0],[-50,50],[-40,0],[-30,-30],[0,40],[30,30])
  Sum : Sum  Inputs=-+  OutDataType=sfix(16)  OutScaling=2^0  SaturateOnIntegerOverflow=on  InputSameDT=on
  dead zone : Constant  Orientation=up  Value=.04  OutDataType=sfix(16)  OutScaling=2^0
  loop breaker : Memory  Orientation=left
  out thresh : Constant  Value=0.2  OutDataType=sfix(16)  OutScaling=2^0
  pgw : Outport  OutDataType=sfix(16)  OutScaling=2^0  InitialOutput=0
  wires:
  Gain/1 -> Sum/1
  loop breaker/1 -> Input Switch/2(pgw)
  Relational Operator2/1 -> Logical Operator/1
  dead zone/1 -> Relational Operator2/2
  Good Reset Integrator1/1(out_1) -> Gain/1
  Logical Operator/1 -> Good Reset Integrator1/2(reset?)
  Sum/1 -> Relational Operator1/1
  PWfn/1 -> Sum/2
  Abs/1 -> Relational Operator2/1, PWfn/1
  Sign/1(out_1) -> loop breaker/1, pgw/1
  mcspl/1 -> Input Switch/1(mcspl)
  Input Switch/1(mcsw) -> Abs/1
  out thresh/1 -> Relational Operator1/2
  Constant1/1 -> Good Reset Integrator1/3(initial condition)
  Constant3/1 -> Good Reset Integrator1/1(input)
  Relational Operator1/1 -> Sign/1(in_1), Logical Operator1/1
  Logical Operator1/1 -> Logical Operator/2

== system pglib/w orig PH table/RefLatch (Default = 50ms) ==
  note: The "NOT" gate outputs a DISABLE signal whenever there is any
      | input, so that there can be no response.
  note: By ANDing these outputs, we get a signal that is DISABLED
      | starting with the beginning of the input pulse, and remains so until
      | rp milliseconds after the termination of the pulse.
  note: The falling edge" block's output becomes DISABLED upon
      | detection of the END of the input pulse, and remains
      | so until the refractory period of rp milliseconds has elapsed.
  note: It's a cheap trick, but it seems to work:
  in_1 : Inport  OutDataType=sfix(16)  OutScaling=2^0
  Abs : Abs  SaturateOnIntegerOverflow=on
  Logical Operator : Logic
  Logical Operator1 : Logic  Operator=NOT  Inputs=1
  trailing edge : Subsystem
      mask Display: disp('Refract\nLatch (te)')
  out_1 : Outport  OutDataType=sfix(16)  OutScaling=2^0  InitialOutput=0
  wires:
  in_1/1 -> Abs/1
  Abs/1 -> trailing edge/1(in_1), Logical Operator1/1
  trailing edge/1(out_1) -> Logical Operator/2
  Logical Operator1/1 -> Logical Operator/1
  Logical Operator/1 -> out_1/1

== system pglib/w orig PH table/SampHold?1 ==
  note: When "S/H?" is HIGH, then "Input" is switched directly to the
      | output ("sample").  When "S/H?" is LOW, the current output is
      | maintained ("hold").
  Input : Inport  OutDataType=sfix(16)  OutScaling=2^0
  S/H? : Inport  Port=2  OutDataType=sfix(16)  OutScaling=2^0
  Memory : Memory  Orientation=left
  Sign : Subsystem
      mask Type: Sign
      mask Description: y = sign(x)
      mask Help: Sign Function:\n\t\t\ty = 1 if x > 0\n\t\t\ty = 0 if x = 0\n\t\t\ty = -1 if x < 0
      mask Display: plot(-50,-50,50,50,[-50,50],[0,0],[0,0],[-50,50],[-40,0],[-30,-30],[0,40],[30,30])
  Switch2 : Switch  Threshold=0.5  SaturateOnIntegerOverflow=on  InputSameDT=on
  output : Outport  OutDataType=sfix(16)  OutScaling=2^0  InitialOutput=0
  wires:
  Memory/1 -> Switch2/3
  Switch2/1 -> Memory/1, output/1
  Input/1 -> Switch2/1
  Sign/1(out_1) -> Switch2/2
  S/H?/1 -> Sign/1(in_1)

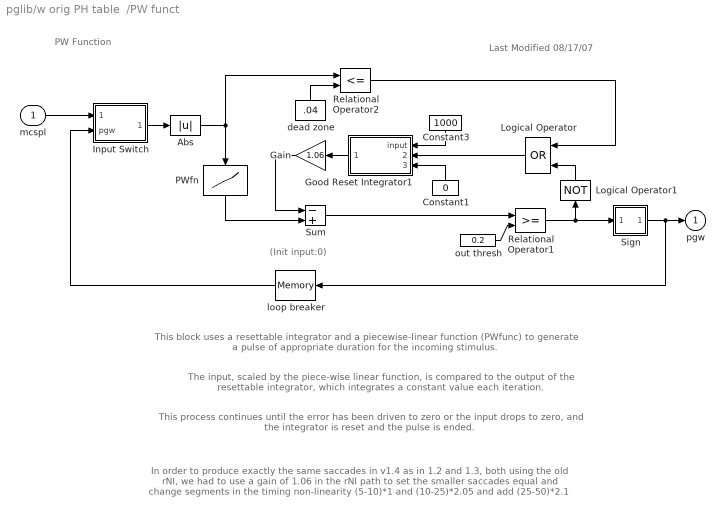
== system pglib/w orig PH table  /PW funct ==
  note: This process continues until the error has been driven to zero or the input drops to zero,
      | and the integrator is reset and the pulse is ended.
  note: The input, scaled by the piece-wise linear function, is compared to the output of the
      | resettable integrator, which integrates a constant value each iteration.
  note: This block uses a resettable integrator and a piecewise-linear function (PWfunc) to generate
      | a pulse of appropriate duration for the incoming stimulus.
  note: (Init input:0)
  note: PW Function
  note: Last Modified
      | 08/17/07
  note: In order to produce exactly the same saccades in v1.4 as in 1.2 and 1.3, both using the old rNI,
      | we had to use a gain of 1.06 in the rNI path to set the smaller saccades equal
      | and change segments in the timing non-linearity (5-10)*1 and  (10-25)*2.05 and add (25-50)*2.1
  mcspl : Inport  OutDataType=sfix(16)  OutScaling=2^0
  Abs : Abs  SaturateOnIntegerOverflow=on
  Constant1 : Constant  Orientation=up  Value=0  OutDataType=sfix(16)  OutScaling=2^0
  Constant3 : Constant  Orientation=down  Value=1000  OutDataType=sfix(16)  OutScaling=2^0
  Gain : Gain  Orientation=left  Gain=1.06  ParameterDataType=sfix(16)  ParameterScaling=2^0  OutDataType=sfix(16)  OutScaling=2^0
  Good Reset Integrator1 : Subsystem  Orientation=left
      mask Display: disp('Resettable\nNI')
  Input Switch : Subsystem
      mask Display: disp('Input\nSwitch')
  Logical Operator : Logic  Orientation=left  Operator=OR
  Logical Operator1 : Logic  Orientation=up  Operator=NOT  Inputs=1
  PWfn : Lookup  Orientation=down  InputValues=[ 0, 0.1:5, 5:10, 10:15, 15:25, 25:50 ]  Table="[ 0, (0.1:5)*0+15,  (5:10)*1+10,  (10:15)*2.0, (15:25)*2.05,  (25:50)*2.1]"  OutDataType=sfix(16)  OutScaling=2^0  SaturateOnIntegerOverflow=on
  Relational Operator1 : RelationalOperator  InputSameDT=on
  Relational Operator2 : RelationalOperator  Operator=<=  InputSameDT=on
  Sign : Subsystem
      mask Type: Sign
      mask Description: y = sign(x)
      mask Help: Sign Function:\n\t\t\ty = 1 if x > 0\n\t\t\ty = 0 if x = 0\n\t\t\ty = -1 if x < 0
      mask Display: plot(-50,-50,50,50,[-50,50],[0,0],[0,0],[-50,50],[-40,0],[-30,-30],[0,40],[30,30])
  Sum : Sum  Inputs=-+  OutDataType=sfix(16)  OutScaling=2^0  SaturateOnIntegerOverflow=on  InputSameDT=on
  dead zone : Constant  Orientation=up  Value=.04  OutDataType=sfix(16)  OutScaling=2^0
  loop breaker : Memory  Orientation=left
  out thresh : Constant  Value=0.2  OutDataType=sfix(16)  OutScaling=2^0
  pgw : Outport  OutDataType=sfix(16)  OutScaling=2^0  InitialOutput=0
  wires:
  Logical Operator1/1 -> Logical Operator/2
  Relational Operator1/1 -> Logical Operator1/1, Sign/1(in_1)
  Constant3/1 -> Good Reset Integrator1/1(input)
  Constant1/1 -> Good Reset Integrator1/3(initial condition)
  out thresh/1 -> Relational Operator1/2
  Input Switch/1(mcsw) -> Abs/1
  mcspl/1 -> Input Switch/1(mcspl)
  Sign/1(out_1) -> pgw/1, loop breaker/1
  Abs/1 -> PWfn/1, Relational Operator2/1
  PWfn/1 -> Sum/2
  Sum/1 -> Relational Operator1/1
  Logical Operator/1 -> Good Reset Integrator1/2(reset?)
  Good Reset Integrator1/1(out_1) -> Gain/1
  dead zone/1 -> Relational Operator2/2
  Relational Operator2/1 -> Logical Operator/1
  loop breaker/1 -> Input Switch/2(pgw)
  Gain/1 -> Sum/1

== system pglib/w orig PH table  /RefLatch (Default = 50ms) ==
  note: It's a cheap trick, but it seems to work:
  note: The falling edge" block's output becomes DISABLED upon
      | detection of the END of the input pulse, and remains
      | so until the refractory period of rp milliseconds has elapsed.
  note: By ANDing these outputs, we get a signal that is DISABLED
      | starting with the beginning of the input pulse, and remains so until
      | rp milliseconds after the termination of the pulse.
  note: The "NOT" gate outputs a DISABLE signal whenever there is any
      | input, so that there can be no response.
  in_1 : Inport  OutDataType=sfix(16)  OutScaling=2^0
  Abs : Abs  SaturateOnIntegerOverflow=on
  Logical Operator : Logic
  Logical Operator1 : Logic  Operator=NOT  Inputs=1
  trailing edge : Subsystem
      mask Display: disp('Refract\nLatch (te)')
  out_1 : Outport  OutDataType=sfix(16)  OutScaling=2^0  InitialOutput=0
  wires:
  Logical Operator/1 -> out_1/1
  Logical Operator1/1 -> Logical Operator/1
  trailing edge/1(out_1) -> Logical Operator/2
  Abs/1 -> Logical Operator1/1, trailing edge/1(in_1)
  in_1/1 -> Abs/1

== system pglib/w orig PH table  /SampHold?1 ==
  note: When "S/H?" is HIGH, then "Input" is switched directly to the
      | output ("sample").  When "S/H?" is LOW, the current output is
      | maintained ("hold").
  Input : Inport  OutDataType=sfix(16)  OutScaling=2^0
  S/H? : Inport  Port=2  OutDataType=sfix(16)  OutScaling=2^0
  Memory : Memory  Orientation=left
  Sign : Subsystem
      mask Type: Sign
      mask Description: y = sign(x)
      mask Help: Sign Function:\n\t\t\ty = 1 if x > 0\n\t\t\ty = 0 if x = 0\n\t\t\ty = -1 if x < 0
      mask Display: plot(-50,-50,50,50,[-50,50],[0,0],[0,0],[-50,50],[-40,0],[-30,-30],[0,40],[30,30])
  Switch2 : Switch  Threshold=0.5  SaturateOnIntegerOverflow=on  InputSameDT=on
  output : Outport  OutDataType=sfix(16)  OutScaling=2^0  InitialOutput=0
  wires:
  S/H?/1 -> Sign/1(in_1)
  Sign/1(out_1) -> Switch2/2
  Input/1 -> Switch2/1
  Switch2/1 -> output/1, Memory/1
  Memory/1 -> Switch2/3
